simulink model "spring_mass_damper"  (R2023b)
settings: Solver=VariableStepAuto  StartTime=0.0  StopTime=300  RelTol=1e-3
settings Model: Creator=farhan  LastModifiedBy=farhan

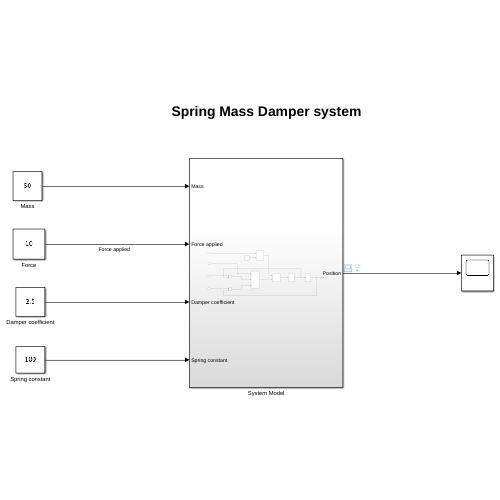
[thumbnail: Simulink's stored preview of the top-level diagram]
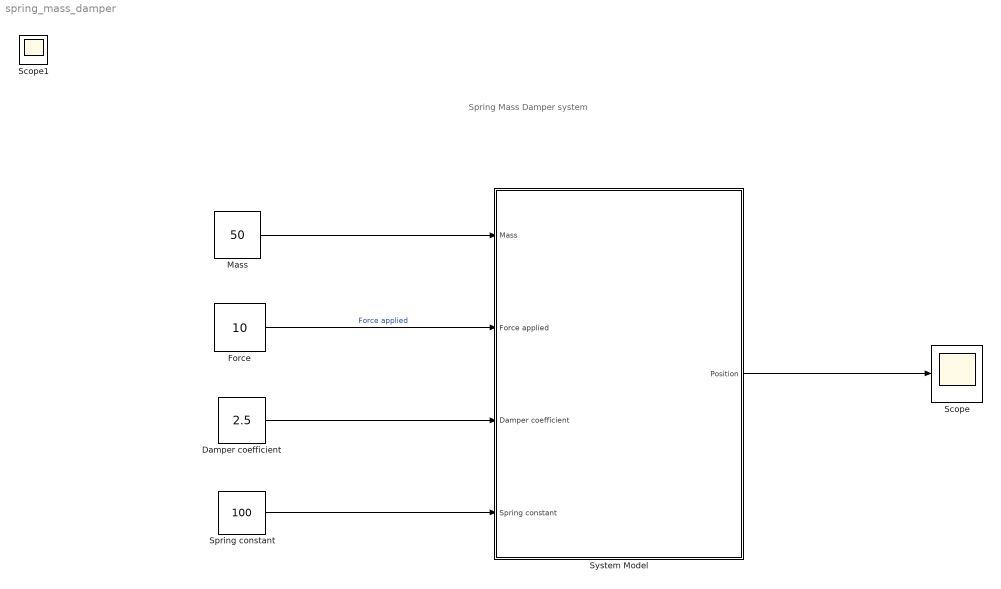
== system spring_mass_damper ==
  note: Spring Mass Damper system
  Damper coefficient : Constant  Value=2.5
  Force : Constant  Value=10
  Mass : Constant  Value=50
  Scope : Scope
  Spring constant : Constant  Value=100
  System Model : Subsystem
  Scope1 : Scope
  wires:
  Mass/1 -> System Model/1(Mass)
  Force/1 -> System Model/2(Force applied)  "Force applied"
  Damper coefficient/1 -> System Model/3(Damper coefficient)
  Spring constant/1 -> System Model/4(Spring constant)
  System Model/1(Position) -> Scope/1

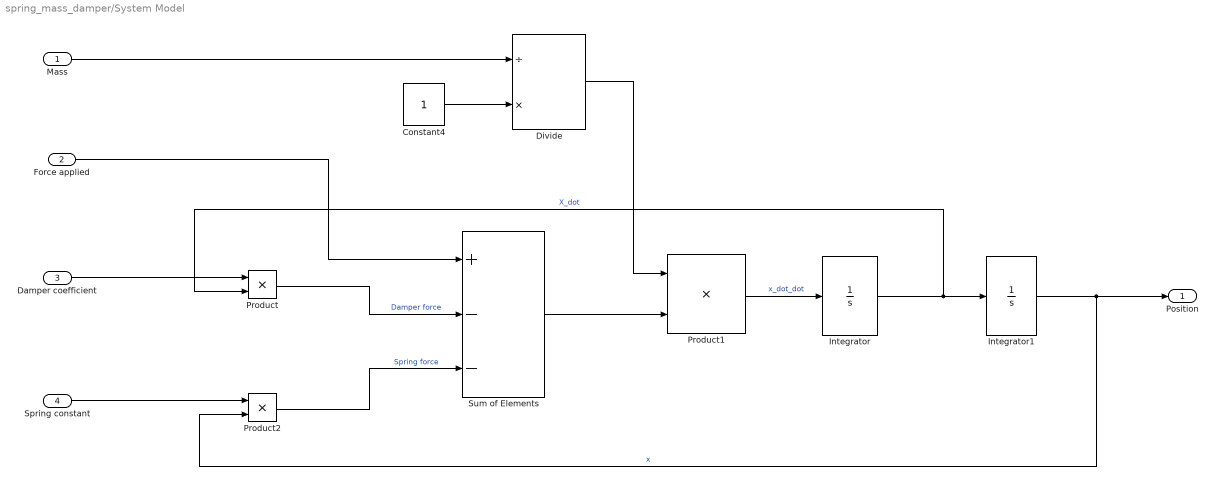
== system spring_mass_damper/System Model ==
  Mass : Inport
  Force applied : Inport  Port=2
  Damper coefficient : Inport  Port=3
  Spring constant : Inport  Port=4
  Constant4 : Constant
  Divide : Product  Inputs=/*
  Integrator : Integrator
  Integrator1 : Integrator
  Product : Product
  Product1 : Product
  Product2 : Product
  Sum of Elements : Sum  Inputs=+--
  Position : Outport
  wires:
  Divide/1 -> Product1/1
  Mass/1 -> Divide/1
  Product/1 -> Sum of Elements/2  "Damper force"
  Sum of Elements/1 -> Product1/2
  Product2/1 -> Sum of Elements/3  "Spring force"
  Integrator/1 -> Product/2, Integrator1/1  "X_dot"
  Integrator1/1 -> Position/1, Product2/2  "x"
  Damper coefficient/1 -> Product/1
  Force applied/1 -> Sum of Elements/1
  Product1/1 -> Integrator/1  "x_dot_dot"
  Constant4/1 -> Divide/2
  Spring constant/1 -> Product2/1
